simulink model "RetourIntegral"  (R2015a)
settings: Solver=ode45  StartTime=0.0  StopTime=10.0  RelTol=1e-5
undefined symbols (not defined in the file or in its folder): CommTD_integral, EE0, EE2, EEIntegral, obsver
settings Model: Creator=Lucien  LastModifiedBy=Lucien

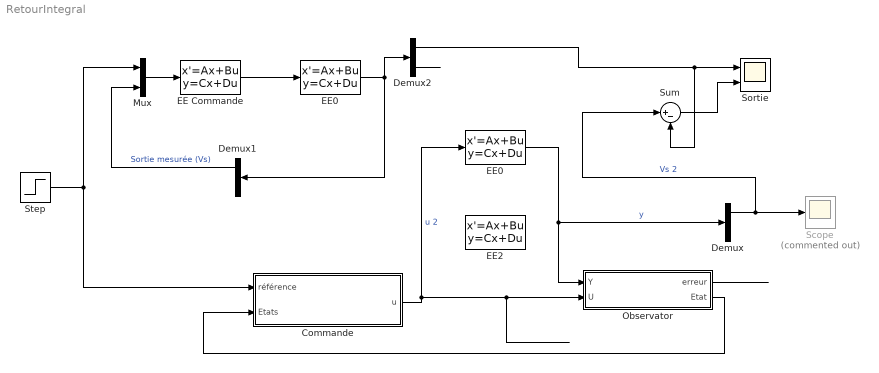
== system RetourIntegral ==
  "Commande " : Subsystem
  Demux : Demux  Outputs=2
  Demux1 : Demux  Outputs=2
  Demux2 : Demux  Outputs=2
  EE Commande : StateSpace  A=CommTD_integral.ee.a  B=CommTD_integral.ee.b  C=CommTD_integral.ee.c  D=CommTD_integral.ee.d  X0=0
  "EE0 " : StateSpace  A=EE0.ee.a  B=EE0.ee.b  C=EE0.ee.c  D=EE0.ee.d  X0=0
  "EE0 " : StateSpace  A=EE0.ee.a  B=EE0.ee.b  C=EE0.ee.c  D=EE0.ee.d  X0=0
  "EE2 " : StateSpace  A=EE2.ee.a  B=EE2.ee.b  C=EE2.ee.c  D=EE2.ee.d  X0=0
  Mux : Mux  Inputs=2
  Observator : Subsystem
  Scope : Scope  Commented=on
      settings: YMin=0.972052  YMax=0.972063  SaveName=ScopeData3
  Sortie : Scope  NumInputPorts=2
      settings: YMin=-5~-5  YMax=5~5  SaveName=ScopeData5
  "Step " : Step  Time=0  SampleTime=0
  Sum : Sum  Inputs=|+-
  wires:
  "EE0 "/1 -> Observator/1("Y "), Demux/1  "y"
  Observator/1(erreur) -> ?
  Demux/1 -> Sum/1, Scope/1  "Vs 2"
  Observator/2("Etat ") -> "Commande "/2(Etats)
  "Commande "/1(u) -> "EE0 "/1, Observator/2(U)  "u 2"
  "Step "/1 -> Mux/1, "Commande "/1(référence)
  EE Commande/1 -> "EE0 "/1
  Mux/1 -> EE Commande/1
  "EE0 "/1 -> Demux2/1, Demux1/1
  Demux1/1 -> Mux/2  "Sortie mesurée (Vs)"
  Demux2/2 -> ?
  Demux2/1 -> Sum/2, Sortie/1
  Sum/1 -> Sortie/2

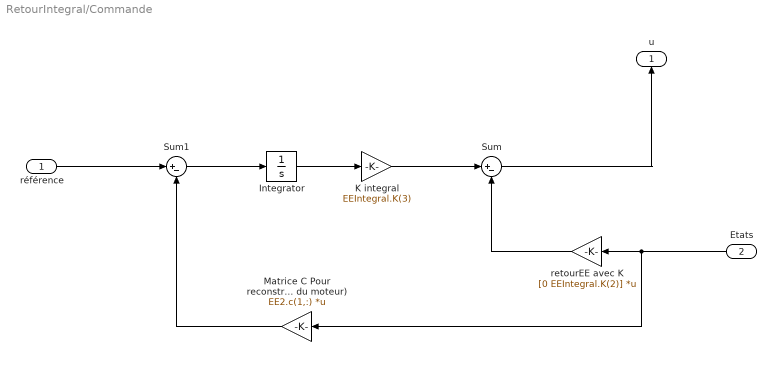
== system RetourIntegral/Commande  ==
  référence : Inport
  Etats : Inport  Port=2
  Integrator : Integrator
  "K integral " : Gain  Gain=EEIntegral.K(3)
  Matrice C Pour reconstruction de Vg(Vitesse du moteur) : Gain  Gain=EE2.c(1,:)  Multiplication=Matrix(K*u)
  Sum : Sum  Inputs=|+-
  Sum1 : Sum  Inputs=|+-
  "retourEE avec K " : Gain  Gain=[0 EEIntegral.K(2)]  Multiplication=Matrix(K*u)
  u : Outport
  wires:
  Sum/1 -> u/1
  "retourEE avec K "/1 -> Sum/2
  "K integral "/1 -> Sum/1
  Sum1/1 -> Integrator/1
  référence/1 -> Sum1/1
  Matrice C Pour reconstruction de Vg(Vitesse du moteur)/1 -> Sum1/2
  Etats/1 -> Matrice C Pour reconstruction de Vg(Vitesse du moteur)/1, "retourEE avec K "/1
  Integrator/1 -> "K integral "/1

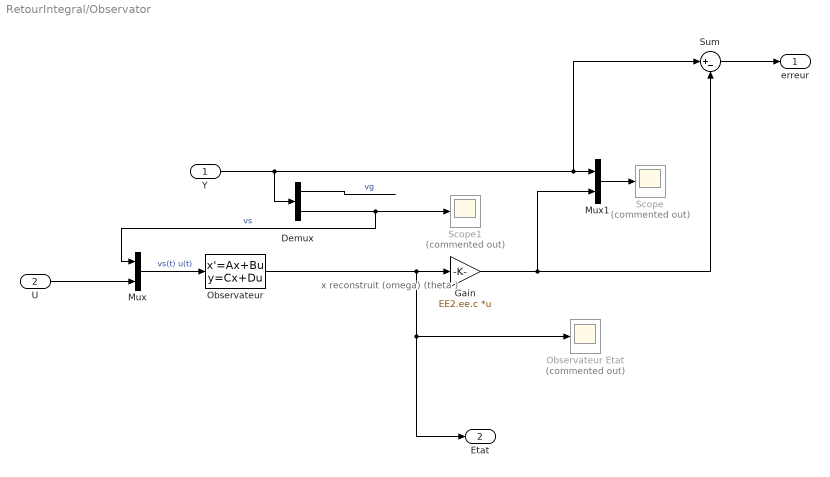
== system RetourIntegral/Observator ==
  note: x reconstruit
      | (omega)
      | (theta   )
  "Y " : Inport
  U : Inport  Port=2
  Demux : Demux  Outputs=2
  Gain : Gain  Gain=EE2.ee.c  Multiplication=Matrix(K*u) (u vector)
  Mux : Mux  Inputs=2
  Mux1 : Mux  Inputs=2
  "Observateur " : StateSpace  A=obsver.ee.a  B=obsver.ee.b  C=obsver.ee.c  D=obsver.ee.d  X0=0
  "Observateur Etat " : Scope  Commented=on
  Scope : Scope  Commented=on
      settings: YMin=-1  YMax=1
  Scope1 : Scope  Commented=on
      settings: YMin=16  YMax=30  SaveName=ScopeData2
  Sum : Sum  Inputs=|+-
  erreur : Outport
  "Etat " : Outport  Port=2
  wires:
  Mux1/1 -> Scope/1
  "Observateur "/1 -> "Etat "/1, "Observateur Etat "/1, Gain/1
  Demux/2 -> Mux/1, Scope1/1  "vs"
  Sum/1 -> erreur/1
  Demux/1 -> ?  "vg"
  "Y "/1 -> Sum/1, Mux1/1, Demux/1
  Mux/1 -> "Observateur "/1  "vs(t) u(t)"
  Gain/1 -> Mux1/2, Sum/2
  U/1 -> Mux/2
